simulink model "pendu_simu"  (R2019b)
settings: Solver=FixedStepAuto  StartTime=0.0  StopTime=10.0  FixedStep=0.01  RelTol=1e-3
values from neighbouring files (symbols this model uses):
  a = 1.42e+01    (= 14.2)    [rotary_ip_lq.m]
  b = 3.45e+00    (= 3.45)    [rotary_ip_lq.m]
  c2 = 3.2973e-04    (= 0.00032973)    [RotatedPendulumParams.m]    (also in ident_pend.m = p2(2); rotary_ip_lq.m = 1.33e-05)
  g = 9.81    [RotatedPendulumParams.m]    (also in ident_pend.m; rotary_ip_lq.m)
  J2b = p2(1)    [ident_pend.m]    (also in rotary_ip_lq.m = 2.9434e-05)
  L1 = 0.265    [RotatedPendulumParams.m]    (also in rotary_ip_lq.m = 0.071)
  l2 = 20e-2    (= 0.2)    [RotatedPendulumParams.m]    (also in ident_pend.m = 0.071; rotary_ip_lq.m = 0.071)
  m2 = 40e-3    (= 0.04)    [RotatedPendulumParams.m]    (also in ident_pend.m = 0.004; rotary_ip_lq.m = 0.004)
undefined symbols (not defined in the file or in its folder): K3
settings Model: Creator=Noritaka Okayasu  LastModifiedBy=Noritaka Okayasu

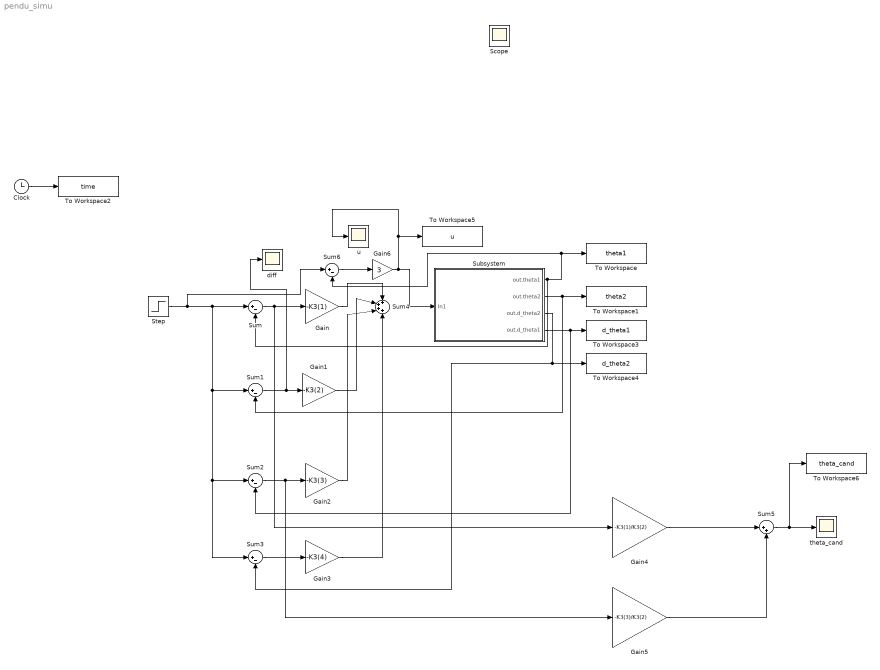
== system pendu_simu ==
  Clock : Clock
  Gain : Gain  Gain=-K3(1)
  Gain1 : Gain  Gain=-K3(2)
  Gain2 : Gain  Gain=-K3(3)
  Gain3 : Gain  Gain=-K3(4)
  Gain4 : Gain  Gain=-K3(1)/K3(2)
  Gain5 : Gain  Gain=-K3(3)/K3(2)
  Gain6 : Gain  Gain=3
  Step : Step  Time=0  After=pi/6  SampleTime=0
  Subsystem : Subsystem
  Sum{,1..3,6} (5 alike) : Sum  Inputs=|+-
  Sum4 : Sum  Inputs=++++
  Sum5 : Sum  Inputs=|++
  To Workspace : ToWorkspace  VariableName=theta1  SampleTime=-1
  To Workspace1 : ToWorkspace  VariableName=theta2  SampleTime=-1
  To Workspace2 : ToWorkspace  VariableName=time  SampleTime=-1
  To Workspace3 : ToWorkspace  VariableName=d_theta1  SaveFormat=Timeseries  SampleTime=-1
  To Workspace4 : ToWorkspace  VariableName=d_theta2  SaveFormat=Timeseries  SampleTime=-1
  To Workspace5 : ToWorkspace  VariableName=u  SaveFormat=Timeseries  SampleTime=-1
  To Workspace6 : ToWorkspace  VariableName=theta_cand  SaveFormat=Timeseries  SampleTime=-1
  diff : Scope
  theta_cand : Scope
  "u " : Scope
  Scope : Scope
  wires:
  Clock/1 -> To Workspace2/1
  Subsystem/1("out.theta1 ") -> To Workspace/1, Sum6/2, Sum/2
  Subsystem/2(out.theta2) -> Sum1/2, To Workspace1/1
  Sum/1 -> Gain4/1, Gain/1
  Step/1 -> Sum6/1, Sum2/1, Sum3/1, Sum1/1, Sum/1
  Subsystem/3(out.d_theta2) -> To Workspace4/1, Sum3/2
  Subsystem/4(out.d_theta1) -> Sum2/2, To Workspace3/1
  Sum1/1 -> diff/1, Gain1/1
  Sum2/1 -> Gain5/1, Gain2/1
  Sum3/1 -> Gain3/1
  Gain1/1 -> Sum4/2
  Gain/1 -> Sum4/1
  Sum5/1 -> To Workspace6/1, theta_cand/1
  Gain4/1 -> Sum5/1
  Gain5/1 -> Sum5/2
  Gain2/1 -> Sum4/3
  Gain3/1 -> Sum4/4
  Gain6/1 -> "u "/1, To Workspace5/1, Subsystem/1(In1)
  Sum6/1 -> Gain6/1

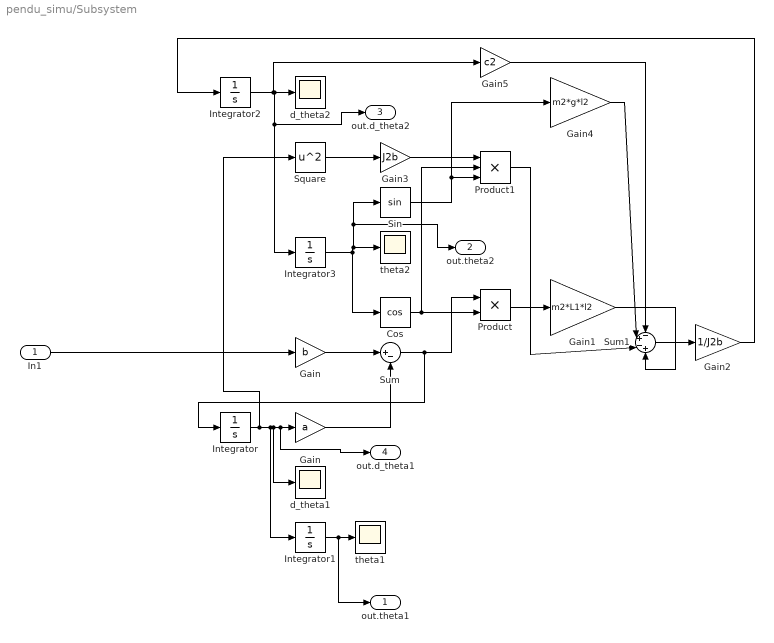
== system pendu_simu/Subsystem ==
  In1 : Inport
  Cos : Trigonometry  Operator=cos
  Gain : Gain  Gain=a
  "Gain " : Gain  Gain=b
  Gain1 : Gain  Gain=m2*L1*l2
  Gain2 : Gain  Gain=1/J2b
  Gain3 : Gain  Gain=J2b
  Gain4 : Gain  Gain=m2*g*l2
  Gain5 : Gain  Gain=c2
  Integrator : Integrator
  Integrator1 : Integrator
  Integrator2 : Integrator
  Integrator3 : Integrator  InitialCondition=pi
  Product : Product
  Product1 : Product  Inputs=3
  Sin : Trigonometry
  Square : Math  Operator=square  SignedPower=off  SaturateOnIntegerOverflow=on
  Sum : Sum  Inputs=|+-
  Sum1 : Sum  Inputs=-+-+
  d_theta1 : Scope
  d_theta2 : Scope
  theta1 : Scope
  theta2 : Scope
  "out.theta1 " : Outport
  out.theta2 : Outport  Port=2
  out.d_theta2 : Outport  Port=3
  out.d_theta1 : Outport  Port=4
  wires:
  Integrator2/1 -> d_theta2/1, out.d_theta2/1, Integrator3/1, Gain5/1
  Integrator/1 -> d_theta1/1, out.d_theta1/1, Gain/1, Integrator1/1, Square/1
  Integrator1/1 -> "out.theta1 "/1, theta1/1
  Gain4/1 -> Sum1/2
  Product1/1 -> Sum1/3
  Integrator3/1 -> theta2/1, out.theta2/1, Sin/1, Cos/1
  "Gain "/1 -> Sum/1
  Sum/1 -> Integrator/1, Product/1
  Gain/1 -> Sum/2
  Sum1/1 -> Gain2/1
  Product/1 -> Gain1/1
  Gain3/1 -> Product1/1
  Sin/1 -> Product1/3, Gain4/1
  Square/1 -> Gain3/1
  In1/1 -> "Gain "/1
  Gain2/1 -> Integrator2/1
  Gain1/1 -> Sum1/4
  Cos/1 -> Product/2, Product1/2
  Gain5/1 -> Sum1/1
